simulink model "sl_puma_hw6"  (R2015a)
settings: Solver=ode45  StartTime=0.0  StopTime=time(end-1)  FixedStep=.001  RelTol=1e-3
values from neighbouring files (symbols this model uses):
  time = [0 0.01 0.02 0.03 0.04 0.05 0.06 0.07 0.08 0.09 0.1 0.11 ... (1001 elements, 1001x1)]    [puma560_torque_profile.mat]
  torque = [2.68302539311e-23 0.0263872953031 0.157921671335 0.31574594673 0.473430845895 0.630698163179 0.787267552104 0.942856958788 1.09718306759 1.24996175724 1.40090856638 1.54973916707 ... (6006 elements, 1001x6)]    [puma560_torque_profile.mat]
libraries: roblocks x2
settings Model: CovSFcnEnable=off  ExtModeTrigMode=oneshot  ExtModeArmWhenConnect=off  Creator=pic  LastModifiedBy=mkillpack
settings DataIOCC: LimitDataPoints=off  SignalLoggingSaveFormat=ModelDataLogs  SignalLogging=off  ReturnWorkspaceOutputs=on
settings OptimizationCC: BlockReduction=off  BooleanDataType=off  ExpressionDepthLimit=2147483647  InitFltsAndDblsToZero=on
settings DebuggingCC: SaveWithParameterizedLinksMsg=none  UnderspecifiedInitializationDetection=Classic  MergeDetectMultiDrivingBlocksExec=none  SignalResolutionControl=TryResolveAllWithWarning  MultiTaskDSMMsg=warning  MultiTaskCondExecSysMsg=none  FcnCallInpInsideContextMsg=EnableAllAsWarning  StateNameClashWarn=warning
settings HardwareCC: TargetUnknown=on
settings GRTTargetCC: ModelReferenceCompliant=off  ParMdlRefBuildCompliant=off  CompOptLevelCompliant=off  CombineOutputUpdateFcns=off  MatFileLogging=off  GRTInterface=on

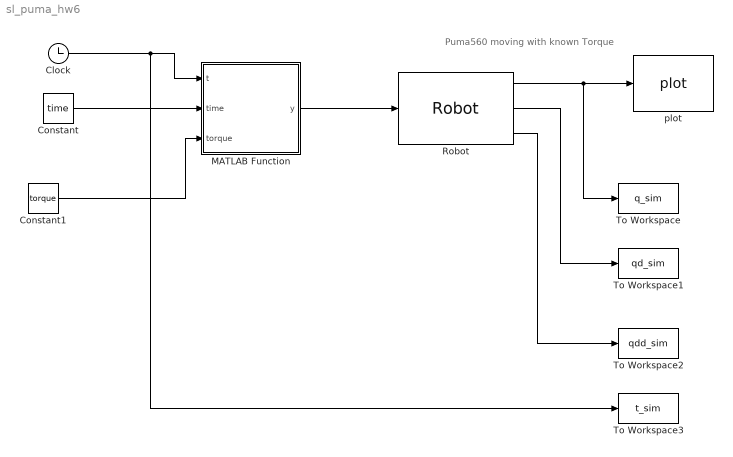
== system sl_puma_hw6 ==
  note: Puma560 moving with known Torque
  Clock : Clock
  Constant : Constant  Value=time
  Constant1 : Constant  Value=torque
  MATLAB Function : MATLAB Function  TreatAsAtomicUnit=on
      settings: PermitHierarchicalResolution=ParametersOnly
  Robot : roblocks/Dynamics/Robot  robot=p560.nofriction  q0=[0 0 0 0 0 0]
  To Workspace : ToWorkspace  VariableName=q_sim  SampleTime=-1
  To Workspace1 : ToWorkspace  VariableName=qd_sim  SampleTime=-1
  To Workspace2 : ToWorkspace  VariableName=qdd_sim  SampleTime=-1
  To Workspace3 : ToWorkspace  VariableName=t_sim  SampleTime=-1
  plot : roblocks/Robot Graphics/plot  robot=p560  fps=25  holdplot=on
  wires:
  Robot/1 -> To Workspace/1, plot/1
  Robot/3 -> To Workspace2/1
  Robot/2 -> To Workspace1/1
  MATLAB Function/1(y) -> Robot/1
  Clock/1 -> To Workspace3/1, MATLAB Function/1(t)
  Constant/1 -> MATLAB Function/2(time)
  Constant1/1 -> MATLAB Function/3(torque)

== matlab function sl_puma_hw6/MATLAB Function ==
  data: t input; y output; time input; torque input
function y = get_torque(t, time, torque)

y = interp1(time, torque, t);

end
